simulink model "regulator_LQ_project"  (R2024a)
settings: Solver=ode45  StartTime=0.0  StopTime=10  RelTol=1e-3  EnableMultiTasking=on
values from neighbouring files (symbols this model uses):
  A = [-Rs/Ld,     we*Lq/Ld ... (first row only)    [project_script.m]    (also in scriptpoint7.m = [-Rs/Ld_real,     we*Lq_real/Ld_real)
  B = [1/Ld,     0 ... (first row only)    [project_script.m]    (also in scriptpoint7.m = [1/Ld_real,     0)
  C = eye(2)    [project_script.m]    (also in scriptpoint7.m)
  D = zeros(2)    [project_script.m]    (also in scriptpoint7.m)
  Ts = 1/8000    (= 0.000125)    [project_script.m]    (also in scriptpoint7.m)
  u_bar_c = -inv(B)*A*xref    [project_script.m]    (also in scriptpoint7.m)
  u_bar_d = Bd\ (eye(size(Ad))-Ad)*xref    [project_script.m]    (also in scriptpoint7.m)
  u_sat_max = [u1_max; u2_max]    [project_script.m]    (also in scriptpoint7.m)
  u_sat_min = [u1_min; u2_min]    [project_script.m]    (also in scriptpoint7.m)
  x0 = [x0_1;x0_2]    [project_script.m]    (also in scriptpoint7.m)
  x_sat_max = [x1_max; x2_max]    [project_script.m]    (also in scriptpoint7.m)
  x_sat_min = [x1_min; x2_min]    [project_script.m]    (also in scriptpoint7.m)
  xref = [6.9; 8.9]    [project_script.m]    (also in scriptpoint7.m)
undefined symbols (not defined in the file or in its folder): Ad, Bd, Cd, Dd, Kc, Kd
settings Model: Creator=Administrator  LastModifiedBy=Utente
settings SolverCC: AlgebraicLoopSolver=TrustRegion
settings DataIOCC: SaveFormat=Array  SignalLoggingSaveFormat=ModelDataLogs  ReturnWorkspaceOutputs=off
settings OptimizationCC: ExpressionDepthLimit=2147483647  InitFltsAndDblsToZero=on  LifeSpan=inf
settings DebuggingCC: UnderspecifiedInitializationDetection=Classic  MergeDetectMultiDrivingBlocksExec=none  SolverPrmCheckMsg=warning  FcnCallInpInsideContextMsg=warning  UnconnectedInputMsg=warning  UnconnectedOutputMsg=warning  UnconnectedLineMsg=warning  StateNameClashWarn=warning  SFUnexpectedBacktrackingDiag=warning  SFNoUnconditionalDefaultTransitionDiag=warning  SFExecutionAtInitializationDiag=none  ArithmeticOperatorsInVariantConditions=warning
settings HardwareCC: ProdBitPerPointer=32  ProdBitPerSizeT=32  ProdBitPerPtrDiffT=32  ProdLargestAtomicFloat=None  ProdIntDivRoundTo=Undefined  ProdEndianess=Unspecified  ProdWordSize=32  ProdHWDeviceType=32-bit Generic
settings ModelReferenceCC: EnableRefExpFcnMdlSchedulingChecks=on  PropagateSignalLabelsOutOfModel=off
settings SFSimCC: SimUseLocalCustomCode=off  CustomCodeUndefinedFunction=UseInterfaceOnly
settings RTWCC: RTWUseLocalCustomCode=off  GPUComputeCapability=3.5
settings CodeAppCC: StateflowObjectComments=on
settings GRTTargetCC: TargetLangStandard=C89/C90 (ANSI)  CombineOutputUpdateFcns=off  GRTInterface=on
settings ConfigComp: CovMetricSettings=dw  CovSaveCumulativeToWorkspaceVar=on  CovSaveSingleToWorkspaceVar=on  CovExternalEMLEnable=off  CovSFcnEnable=off

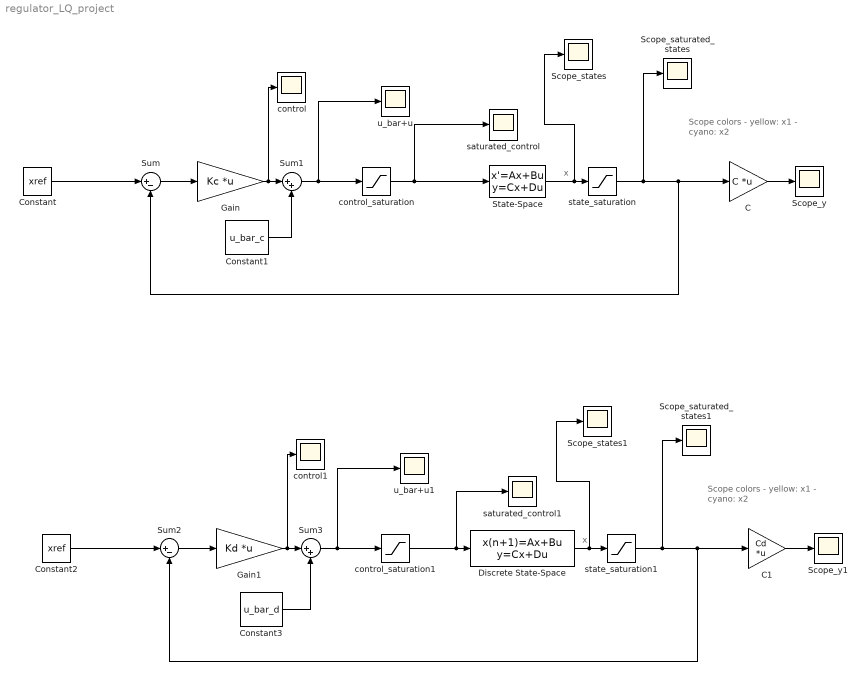
== system regulator_LQ_project ==
  note: x
  note: Scope colors
      | - yellow: x1
      | - cyano: x2
  note: x
  note: Scope colors
      | - yellow: x1
      | - cyano: x2
  C : Gain  Gain=C  Multiplication=Matrix(K*u)
  C1 : Gain  Gain=Cd  Multiplication=Matrix(K*u)
  Constant : Constant  Value=xref
  Constant1 : Constant  Value=u_bar_c
  Constant2 : Constant  Value=xref  SampleTime=Ts
  Constant3 : Constant  Value=u_bar_d  SampleTime=Ts
  Discrete State-Space : DiscreteStateSpace  A=Ad  B=Bd  C=Cd  D=Dd  InitialCondition=x0  SampleTime=Ts
  Gain : Gain  Gain=Kc  Multiplication=Matrix(K*u)
  Gain1 : Gain  Gain=Kd  Multiplication=Matrix(K*u)
  Scope_saturated_states : Scope
  Scope_saturated_states1 : Scope
  Scope_states : Scope
  Scope_states1 : Scope
  Scope_y : Scope
  Scope_y1 : Scope
  "State-Space " : StateSpace  A=A  B=B  C=C  D=D  InitialCondition=x0
  Sum : Sum  Inputs=|+-
  Sum1 : Sum  Inputs=|++
  Sum2 : Sum  Inputs=|+-
  Sum3 : Sum  Inputs=|++
  control : Scope
  control1 : Scope
  control_saturation : Saturate  UpperLimit=u_sat_max  LowerLimit=u_sat_min
  control_saturation1 : Saturate  UpperLimit=u_sat_max  LowerLimit=u_sat_min
  saturated_control : Scope
  saturated_control1 : Scope
  state_saturation : Saturate  UpperLimit=x_sat_max  LowerLimit=x_sat_min
  state_saturation1 : Saturate  UpperLimit=x_sat_max  LowerLimit=x_sat_min
  u_bar+u : Scope
  u_bar+u1 : Scope
  wires:
  control_saturation/1 -> "State-Space "/1, saturated_control/1
  Sum/1 -> Gain/1
  "State-Space "/1 -> Scope_states/1, state_saturation/1
  C/1 -> Scope_y/1
  Constant/1 -> Sum/1
  Gain/1 -> control/1, Sum1/1
  Constant1/1 -> Sum1/2
  Sum1/1 -> control_saturation/1, u_bar+u/1
  state_saturation/1 -> Sum/2, C/1, Scope_saturated_states/1
  Constant2/1 -> Sum2/1
  Gain1/1 -> control1/1, Sum3/1
  Sum2/1 -> Gain1/1
  state_saturation1/1 -> Sum2/2, C1/1, Scope_saturated_states1/1
  Sum3/1 -> control_saturation1/1, u_bar+u1/1
  C1/1 -> Scope_y1/1
  Constant3/1 -> Sum3/2
  Discrete State-Space/1 -> Scope_states1/1, state_saturation1/1
  control_saturation1/1 -> saturated_control1/1, Discrete State-Space/1
